simulink model "sistema"  (R2023a)
settings: Solver=ode23t  StartTime=0.0  StopTime=10.0  RelTol=1e-3
libraries: fl_lib x8, nesl_utility x3, ee_lib x1, slpidlib x1, simulink x1
settings Model: Creator=vanes  LastModifiedBy=vanes
settings DebuggingCC: AlgebraicLoopMsg=none  ArtificialAlgebraicLoopMsg=none  MaxConsecutiveZCsMsg=none  ModelReferenceExtraNoncontSigs=none  OperatingPointInterfaceChecksumMismatchMsg=none

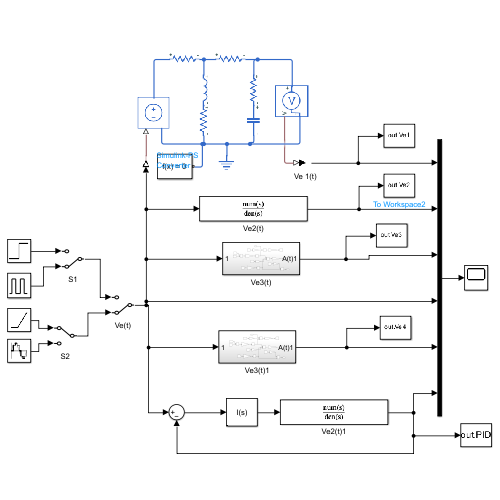
[thumbnail: Simulink's stored preview of the top-level diagram]
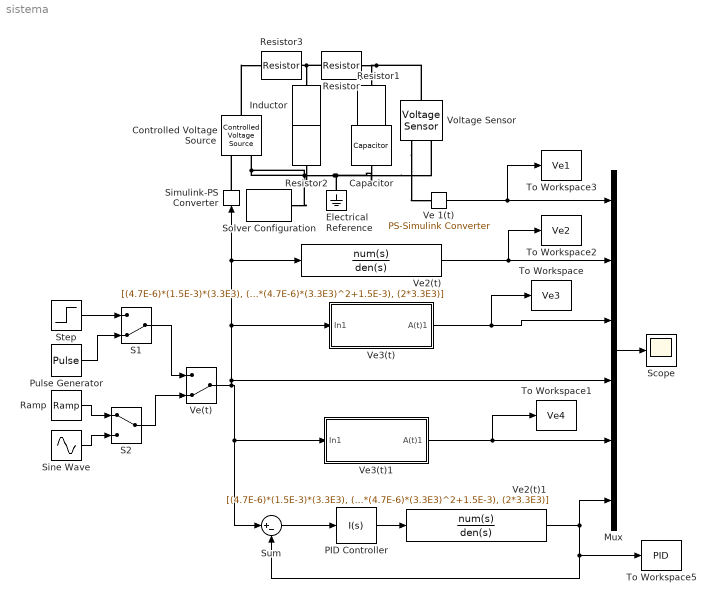
== system sistema ==
  Capacitor : ee_lib/Passive/Capacitor  cap_option=ee.enum.passive.capacitor.capOption.const  c=47e-5 F  Cvec=[1e-05, 1e-06] F  Vvec=[0, 10] V  CV_table_symmetry=ee.enum.passive.capacitor.tableSymmetry.yes  f_vec=[1, 10] kHz  DFext_vec=[.8, 1.2]  enable_C_tol=ee.enum.toleranceApplication.none  averaging_period=0 s  C_tol=5  tol_distribution=ee.enum.toleranceDistribution.uniform  nSigma=4  r=1e-6 Ohm  g=0 1/Ohm  enable_operating_limits=ee.enum.enable.no  enable_faults=ee.enum.enable.no  fault_action=simscape.enum.assert.action.none  Cscale_faulted=100  R_faulted=1e-3 Ohm  G_faulted=0 1/Ohm  tau_fault=1e-3 s  fault_trigger=ee.enum.faults.faultTrigger.temporal  t_fault=1 s  max_permissible_voltage_range=[-100, 100] V  t_fail_on_voltage=1 s  operating_limit_action=ee.enum.passive.reportOpLim.warn  max_working_voltage_range=[-25, 25] V  power_rating=1 W  i_specify=off  i_priority=None  i=0 A  i_nominal_specify=off  i_nominal_unit=A  i_nominal_value=1  v_specify=off  v_priority=None  v=0 V  v_nominal_specify=off  v_nominal_unit=V  v_nominal_value=1  vc_specify=off  vc_priority=High  vc=0 V  vc_nominal_specify=off  vc_nominal_unit=V  vc_nominal_value=1
  Controlled Voltage Source : fl_lib/Electrical/Electrical Sources/Controlled Voltage Source
  Electrical Reference : fl_lib/Electrical/Electrical Elements/Electrical Reference
  Inductor : fl_lib/Electrical/Electrical Elements/Inductor  l=1.5e-3 H  r=0 Ohm  g=1e-9 1/Ohm  i_specify=off  i_priority=None  i=0 A  i_nominal_specify=off  i_nominal_unit=A  i_nominal_value=1  v_specify=off  v_priority=None  v=0 V  v_nominal_specify=off  v_nominal_unit=V  v_nominal_value=1  i_L_specify=off  i_L_priority=High  i_L=0 A  i_L_nominal_specify=off  i_L_nominal_unit=A  i_L_nominal_value=1
  Mux : Mux  Inputs=6
  PID Controller : slpidlib/PID Controller  Controller=I  Form=Parallel  TimeDomain=Continuous-time  UseExternalTs=off  SampleTime=-1  IntegratorMethod=Forward Euler  FilterMethod=Forward Euler  ControllerParametersSource=internal  P=0  I=5826.83507312895  UseKiTs=off  D=0  N=100  UseFilter=on  TunerSelectOption=Transfer Function Based (PID Tuner App)  InitialConditionSource=internal  InitialConditionForIntegrator=0  InitialConditionForFilter=0  DifferentiatorICPrevScaledInput=0  ExternalReset=none  TrackingMode=off  Kt=1  LimitOutput=off  SatLimitsSource=internal  UpperSaturationLimit=inf  LowerSaturationLimit=-inf  LinearizeAsGain=on  AntiWindupMode=none  Kb=1  LimitIntegrator=off  UpperIntegratorSaturationLimit=inf  LowerIntegratorSaturationLimit=-inf  POutMin=[]  POutMax=[]  IOutMin=[]  IOutMax=[]  DOutMin=[]  DOutMax=[]  NOutMin=[]  NOutMax=[]  SumOutMin=[]  SumOutMax=[]  SaturationOutMin=[]  SaturationOutMax=[]  PParamMin=[]  PParamMax=[]  IParamMin=[]  IParamMax=[]  DParamMin=[]  DParamMax=[]  NParamMin=[]  NParamMax=[]  KbParamMin=[]  KbParamMax=[]  KtParamMin=[]  KtParamMax=[]  KbOutMin=[]  KbOutMax=[]  KtOutMin=[]  KtOutMax=[]  IntegratorOutMin=[]  IntegratorOutMax=[]  FilterOutMin=[]  FilterOutMax=[]  SumI1OutMin=[]  SumI1OutMax=[]  SumI2OutMin=[]  SumI2OutMax=[]  SumI3OutMin=[]  SumI3OutMax=[]  SumI4OutMin=[]  SumI4OutMax=[]  SumDOutMin=[]  SumDOutMax=[]  DifferentiatorOutMin=[]  DifferentiatorOutMax=[]  FilterDiffOutCoefMin=[]  FilterDiffOutCoefMax=[]  ReciprocalOutMin=[]  ReciprocalOutMax=[]  SumDenOutMin=[]  SumDenOutMax=[]  SumNumOutMin=[]  SumNumOutMax=[]  DivideOutMin=[]  DivideOutMax=[]  UdiffTsProdOutMin=[]  UdiffTsProdOutMax=[]  NTsProdOutMin=[]  NTsProdOutMax=[]  UintegralTsProdOutMin=[]  UintegralTsProdOutMax=[]  UngainTsProdOutMin=[]  UngainTsProdOutMax=[]  ClampingZeroOutDataTypeStr=Inherit: Inherit via back propagation  ClampingZeroOutMin=[]  ClampingZeroOutMax=[]  FilterDenConstantOutDataTypeStr=Inherit: Inherit via back propagation  FilterDenConstantOutMin=[]  FilterDenConstantOutMax=[]  PCopyOutDataTypeStr=Inherit: Inherit via back propagation  PCopyOutMin=[]  PCopyOutMax=[]  NCopyOutDataTypeStr=Inherit: Inherit via back propagation  NCopyOutMin=[]  NCopyOutMax=[]  IntegratorContinuousStateAttributes=''  IntegratorStateMustResolveToSignalObject=off  IntegratorRTWStateStorageClass=Auto  FilterContinuousStateAttributes=''  FilterStateMustResolveToSignalObject=off  FilterRTWStateStorageClass=Auto  ParallelPVariant=Disabled  IdealPVariant=Disabled  IVariant=InternalParameters  DVariant=Disabled  IntegratorVariant=Continuous  SatVariant=Disabled  AWVariant=Passthrough  PCopyVariant=Disabled  TRVariant=Disabled  FdbkBlocksVariant=Forward  IdealPFdbkVariant=Disabled  SatFdbkVariant=Disabled  DerivativeFilterVariant=Disabled  NVariant=Disabled  NCopyVariant=Disabled_SignalSpec  FilterICVariant=Disabled  IntegratorICVariant=InternalICs  ExternalResetVariant=Disabled  TRSumVariant=Passthrough  SumFdbkVariant=Disabled  SumVariant=Passthrough_I  TsampFilterVariant=InternalTs  TsampNgainVariant=Passthrough  TsampIntegralVariant=Disabled_SignalSpec  ExternalSaturationOutDataTypeStr=Inherit: Same as second input
  Pulse Generator : DiscretePulseGenerator  PulseType=Time based  Period=10  PulseWidth=10  PhaseDelay=1
  Ramp : simulink/Sources/Ramp  slope=1/10  start=0  InitialOutput=0
  Resistor{,1..3} (4 alike) : fl_lib/Electrical/Electrical Elements/Resistor  R=3300 Ohm  i_specify=off  i_priority=None  i=0 A  i_nominal_specify=off  i_nominal_unit=A  i_nominal_value=1  v_specify=off  v_priority=None  v=0 V  v_nominal_specify=off  v_nominal_unit=V  v_nominal_value=1
  S1 : ManualSwitch  CurrentSetting=0
  S2 : ManualSwitch
  Scope : Scope
  Simulink-PS Converter : nesl_utility/Simulink-PS Converter  PhysicalDomain=network_engine_domain  SubClassName=ps_input  LeftPortType=input  RightPortType=output  PseudoPeriodic=off  Frequencies=[]  NoiseDistribution=none  NoiseParameters=[]  Unit=1  AffineConversion=off  FilteringAndDerivatives=provide  SimscapeFilterOrder=1  InputFilterTimeConstant=0.001  UdotUserProvided=0
  Sine Wave : Sin  Frequency=pi/2  SampleTime=0.01
  Solver Configuration : nesl_utility/Solver Configuration  PhysicalDomain=network_engine_domain  SubClassName=solver  LeftPortType=input  RightPortType=generic  Tones=[]  Harmonics=[]  SimulateNoise=off  Profile=off  UseLocalSampling=off  EnableSwitchedLinearOptims=on  FrequencyDomain=off  UseCCode=off  RelTol=0.001  AbsTol=0.001  MinStep=1e-09  ToWorkspace=off  RevertToSquareIcSolve=off  NumHomotopyIterations=100  PhasorMode=off  PhasorModeNumHarmonics=1  ConsistencySolver=NEWTON_XTOL_AFTER_FTOL  IndexReductionMethod=DerivativeReplacement  DoDC=off  ResidualTolerance=1e-09  ConsistencyTolSource=GLOBAL  ConsistencyAbsTol=0.001  ConsistencyRelTol=0.001  ConsistencyTolFactor=0.001  UseLocalSolver=off  LocalSolverChoice=NE_BACKWARD_EULER_ADVANCER  ResolveIndetEquations=on  FunctionEvalNumThread=1  LocalSolverSampleTime=0.001  DoFixedCost=off  MaxNonlinIter=3  MaxModeIter=2  ComputeImpulses=off  ImpulseIterations=2  LinearAlgebra=auto  LinearAlgebraNumThread=0  EquationFormulation=NE_TIME_EF  DelaysMemoryBudget=1024  AutomaticFiltering=on  FilteringTimeConstant=0.001  PartitionStorageMethod=AS_NEEDED  PartitionMemoryBudget=1024  PartitionMethod=ROBUST
  Step : Step  Time=0  SampleTime=0.001
  Sum : Sum  Inputs=|+-
  To Workspace : ToWorkspace  VariableName=Ve3  SampleTime=-1
  To Workspace1 : ToWorkspace  VariableName=Ve4  SampleTime=-1
  To Workspace2 : ToWorkspace  VariableName=Ve2  SampleTime=-1
  To Workspace3 : ToWorkspace  VariableName=Ve1  SampleTime=-1
  To Workspace5 : ToWorkspace  VariableName=PID  SampleTime=-1
  Ve 1(t) : nesl_utility/PS-Simulink Converter  PhysicalDomain=network_engine_domain  SubClassName=ps_output  LeftPortType=input  RightPortType=output  PseudoPeriodic=off  Frequencies=[]  VectorFormat=1-D array  Unit=inherit  AffineConversion=off
  Ve(t) : ManualSwitch  CurrentSetting=0
  Ve2(t) : TransferFcn  Numerator=[(4.7E-6)*(1.5E-3)*(3.3E3), ((4.7E-6)*(3.3E3)^2+1.5E-3), 3.3E3]  Denominator=[3*(4.7E-6)*(1.5E-3)*(3.3E3), (5*(4.7E-6)*(3.3E3)^2+1.5E-3), (2*3.3E3)]
  Ve2(t)1 : TransferFcn  Numerator=[(4.7E-6)*(1.5E-3)*(3.3E3), ((4.7E-6)*(3.3E3)^2+1.5E-3), 3.3E3]  Denominator=[3*(4.7E-6)*(1.5E-3)*(3.3E3), (5*(4.7E-6)*(3.3E3)^2+1.5E-3), (2*3.3E3)]
  Ve3(t) : Subsystem
  Ve3(t)1 : Subsystem
  Voltage Sensor : fl_lib/Electrical/Electrical Sensors/Voltage Sensor
  wires:
  Mux/1 -> Scope/1
  Sine Wave/1 -> S2/2
  Sum/1 -> PID Controller/1
  Ramp/1 -> S2/1
  Pulse Generator/1 -> S1/2
  Step/1 -> S1/1
  Ve(t)/1 -> Sum/1, Ve3(t)1/1(In1), Ve2(t)/1, Simulink-PS Converter/1, Ve3(t)/1(In1), Mux/4
  S2/1 -> Ve(t)/2
  S1/1 -> Ve(t)/1
  Ve 1(t)/1 -> To Workspace3/1, Mux/1
  Ve2(t)/1 -> To Workspace2/1, Mux/2
  Ve3(t)/1(A(t)1) -> To Workspace/1, Mux/3
  Ve3(t)1/1(A(t)1) -> To Workspace1/1, Mux/5
  PID Controller/1 -> Ve2(t)1/1
  Ve2(t)1/1 -> To Workspace5/1, Sum/2, Mux/6
  connections:
  Voltage Sensor/LConn1 -- Resistor1/LConn1 -- Resistor/RConn1
  Resistor/LConn1 -- Resistor3/RConn1 -- Inductor/LConn1
  Controlled Voltage Source/RConn2 -- Solver Configuration/RConn1 -- Resistor2/RConn1 -- Voltage Sensor/RConn2 -- Capacitor/RConn1 -- Electrical Reference/LConn1
  Inductor/RConn1 -- Resistor2/LConn1
  Voltage Sensor/RConn1 -- Ve 1(t)/LConn1
  Simulink-PS Converter/RConn1 -- Controlled Voltage Source/RConn1
  Resistor1/RConn1 -- Capacitor/LConn1
  Controlled Voltage Source/LConn1 -- Resistor3/LConn1

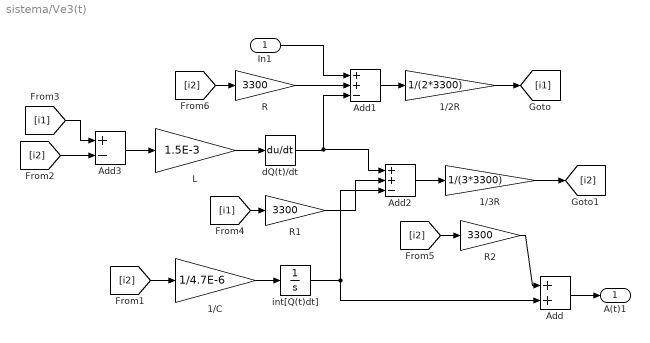
== system sistema/Ve3(t) ==
  In1 : Inport
  1/2R : Gain  Gain=1/(2*3300)
  1/3R : Gain  Gain=1/(3*3300)
  1/C : Gain  Gain=1/4.7E-6
  Add : Sum
  Add1 : Sum  Inputs=++-
  Add2 : Sum  Inputs=++-
  Add3 : Sum  Inputs=+-
  L : Gain  Gain=1.5E-3
  R : Gain  Gain=3300
  R1 : Gain  Gain=3300
  R2 : Gain  Gain=3300
  dQ(t)/dt : Derivative
  int[Q(t)dt] : Integrator
  A(t)1 : Outport
  wires:
  1/2R/1 -> [i1]
  [i2] -> 1/C/1
  [i2] -> R/1
  R/1 -> Add1/2
  Add1/1 -> 1/2R/1
  1/3R/1 -> [i2]
  dQ(t)/dt/1 -> Add1/3, Add2/1
  L/1 -> dQ(t)/dt/1
  Add2/1 -> 1/3R/1
  Add3/1 -> L/1
  [i2] -> Add3/2
  [i1] -> Add3/1
  R1/1 -> Add2/2
  [i1] -> R1/1
  1/C/1 -> int[Q(t)dt]/1
  int[Q(t)dt]/1 -> Add2/3, Add/2
  [i2] -> R2/1
  In1/1 -> Add1/1
  R2/1 -> Add/1
  Add/1 -> A(t)1/1

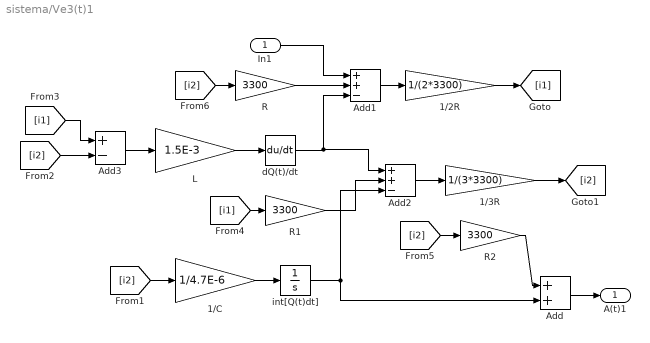
== system sistema/Ve3(t)1 ==
  In1 : Inport
  1/2R : Gain  Gain=1/(2*3300)
  1/3R : Gain  Gain=1/(3*3300)
  1/C : Gain  Gain=1/4.7E-6
  Add : Sum
  Add1 : Sum  Inputs=++-
  Add2 : Sum  Inputs=++-
  Add3 : Sum  Inputs=+-
  L : Gain  Gain=1.5E-3
  R : Gain  Gain=3300
  R1 : Gain  Gain=3300
  R2 : Gain  Gain=3300
  dQ(t)/dt : Derivative
  int[Q(t)dt] : Integrator
  A(t)1 : Outport
  wires:
  1/2R/1 -> [i1]
  [i2] -> 1/C/1
  [i2] -> R/1
  R/1 -> Add1/2
  Add1/1 -> 1/2R/1
  1/3R/1 -> [i2]
  dQ(t)/dt/1 -> Add1/3, Add2/1
  L/1 -> dQ(t)/dt/1
  Add2/1 -> 1/3R/1
  Add3/1 -> L/1
  [i2] -> Add3/2
  [i1] -> Add3/1
  R1/1 -> Add2/2
  [i1] -> R1/1
  1/C/1 -> int[Q(t)dt]/1
  int[Q(t)dt]/1 -> Add2/3, Add/2
  [i2] -> R2/1
  In1/1 -> Add1/1
  R2/1 -> Add/1
  Add/1 -> A(t)1/1
